simulink model "Q6_SIM"  (R2024b)
settings: Solver=VariableStepAuto  StartTime=0.0  StopTime=10.0  RelTol=1e-3
values from neighbouring files (symbols this model uses):
  D = zeros(2,1)    [main.m]
  K = lqr(A, B, Qr, Rr)    [IP_MACRO.m]    (also in main_sim.m = lqr(A_aug, B_aug, Qr, Rr))
  x0 = [alpha_init 0 beta_init 0 0]'    [main.m]    (also in main_sim.m = [alpha_init 0 beta_init 0 0])
undefined symbols (not defined in the file or in its folder): A, B
settings Model: Creator=pedro  LastModifiedBy=pedro

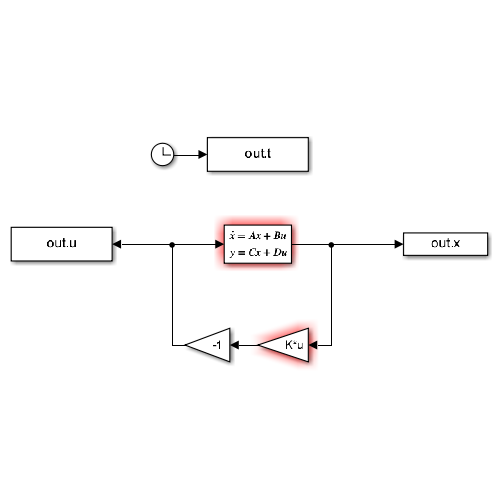
[thumbnail: Simulink's stored preview of the top-level diagram]
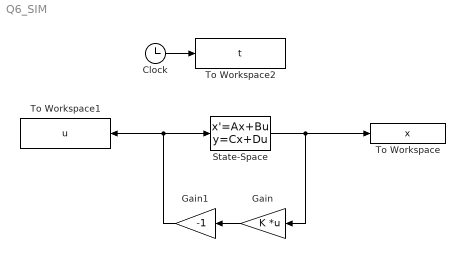
== system Q6_SIM ==
  Clock : Clock
  Gain : Gain  Gain=K  Multiplication=Matrix(K*u)
  Gain1 : Gain  Gain=-1
  State-Space : StateSpace  A=A  B=B  C=eye(5)  D=D  InitialCondition=x0  ContinuousStateAttributes={'x1','x2','x3','x4','x5'}
  To Workspace : ToWorkspace  VariableName=x  SaveFormat=Timeseries  SampleTime=-1
  To Workspace1 : ToWorkspace  VariableName=u  SaveFormat=Timeseries  SampleTime=-1
  To Workspace2 : ToWorkspace  VariableName=t  SaveFormat=Timeseries  SampleTime=-1
  wires:
  State-Space/1 -> To Workspace/1, Gain/1
  Clock/1 -> To Workspace2/1
  Gain/1 -> Gain1/1
  Gain1/1 -> To Workspace1/1, State-Space/1
